simulink model "playback_data"  (R2015a)
settings: Solver=FixedStepDiscrete  SolverMode=SingleTasking  StartTime=44  StopTime=72  FixedStep=sample_time  RelTol=1e-3
undefined symbols (not defined in the file or in its folder): A_kalman_no_position, A_kalman_transverse, A_kalman_vertical, A_lpf_10hz_05d, A_lpf_accelerometer, A_lpf_fourbar_angles, A_lpf_imu, A_lpf_lateral_angle, B1_lpf_10hz_05d, B1_lpf_accelerometer, B1_lpf_fourbar_angles, B1_lpf_imu, B1_lpf_lateral_angle, B2_lpf_10hz_05d, B2_lpf_accelerometer, B2_lpf_fourbar_angles, B2_lpf_imu, B2_lpf_lateral_angle, B_dx_versus_x0, B_kalman_no_position, B_kalman_transverse, B_kalman_vertical, backwards_K_sag_of_t, backwards_P_sag_of_t, boom_mount_angle, C_kalman_no_position, C_kalman_transverse, C_kalman_vertical, com_leg_motor, com_torso, contact_threshold, control_start_time, d_ankle_to_foot, d_vertical_boom_com_offset, d_vertical_com, desired_com_forward_velocity, desired_com_lateral_velocity, desired_initial_leg_roll_left, desired_initial_leg_roll_right, desired_standing_torso_pitch, desired_standing_torso_roll, desired_standing_z, desired_torso_pitch, desired_torso_roll, Discrete, enable_bouncing, fcut_contact, fdesignblkfcn, forward_dx_of_dxstar, forward_x_of_dxstar, g, gcbh, h_boom, HIP_MTR_MAX_CONT_TORQUE, HIP_MTR_MAX_TORQUE, i_leg_motor, i_robot, i_torso, initial_dx_estimate, initial_dx_takeoff_history ... (+82)
libraries: simulink x23, ctrlSharedLib x4, dsparch4 x3, dspfdesign x1
(part 3 of 6)

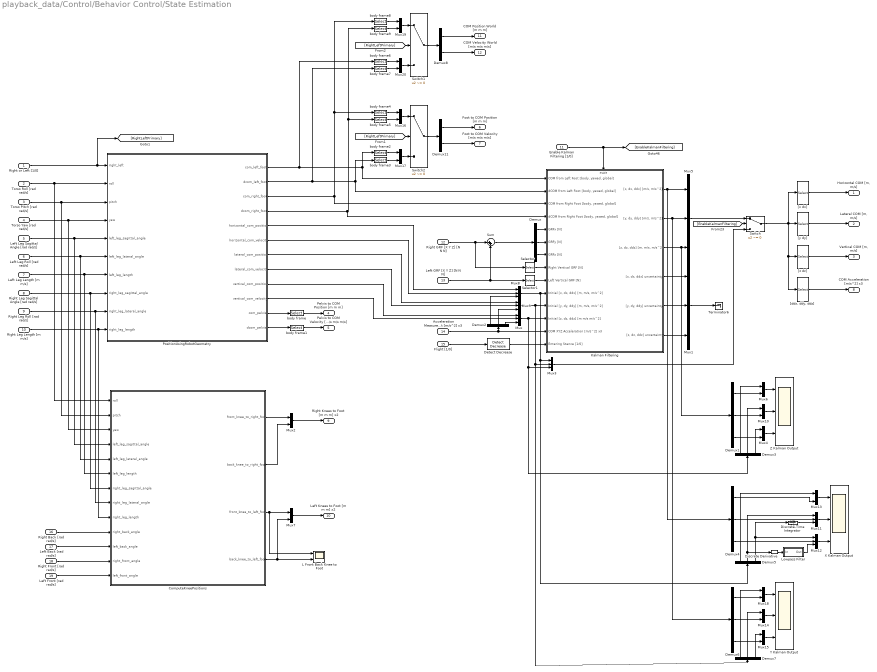
== system playback_data/Control/Behavior Control/State Estimation ==
  Right or Left [1/0] : Inport
  Torso Roll [rad rad/s] : Inport  Port=2
  Torso Pitch [rad rad/s] : Inport  Port=3
  Torso Yaw [rad rad/s] : Inport  Port=4
  Left Leg Sagittal Angle [rad rad/s] : Inport  Port=5
  Left Leg Roll [rad rad/s] : Inport  Port=6
  Left Leg Length [m m/s] : Inport  Port=7
  Right Leg Sagittal Angle [rad rad/s] : Inport  Port=8
  Right Leg Roll [rad rad/s] : Inport  Port=9
  Right Leg Length [m m/s] : Inport  Port=10
  Enable Kalman Filtering [1/0] : Inport  Port=11
  Right GRF [X Y Z] [N N N] : Inport  Port=12
  Left GRF [X Y Z] [N N N] : Inport  Port=13
  " Acceleration Measurement [m/s^2] x3" : Inport  Port=14
  Flight [1/0] : Inport  Port=15
  Right Back [rad rad/s] : Inport  Port=16
  Left Back [rad rad/s] : Inport  Port=17
  Right Front [rad rad/s] : Inport  Port=18
  Left Front [rad rad/s] : Inport  Port=19
  ComputeKneePositions : MATLAB Function  TreatAsAtomicUnit=on
  Demux{,1..7} (8 alike) : Demux  Outputs=3
  Demux11 : Demux  Outputs=2
  Demux8 : Demux  Outputs=2
  Detect Decrease : simulink/Logic and Bit Operations/Detect Decrease  vinit=0.0  InputProcessing=Inherited  OutDataTypeStr=boolean
  Discrete Derivative : simulink/Discrete/Discrete Derivative  gainval=1.0  ICPrevScaledInput=0.0  InputProcessing=Inherited  OutMin=[]  OutMax=[]  OutDataType=fixdt(1, 16)  OutScaling=2^-10  DoSatur=off
  Discrete-Time Integrator : DiscreteIntegrator  InitialConditionSetting=State (most efficient)  SampleTime=-1
  Kalman Filtering : Subsystem
  L Front Back Knee to Foot : Scope  NumInputPorts=2
      settings: YMin=-0.425~-0.5  YMax=-0.025~0.3  SaveName=ScopeData44  SampleInput=on
  Lowpass Filter : Subsystem  DialogController=fdesignblkfcn  InitFcn=fdesignblkfcn(gcbh, {'InitFcn'});  mask(Lowpass Filter){}
      mask help: Design a lowpass filter
      settings: CopyFcn=fdesignblkfcn(gcbh, {'CopyFcn'});
      mask Help: helpview(mapfilelocation('dsp'), 'dsplowpassfilter');
      mask Display: disp('Lowpass')
  Mux{,1,3,5,8..9,11..12} (8 alike) : Mux  Inputs=3
  Mux{2,4,6..7,10,13..20} (13 alike) : Mux  Inputs=2
  PositionUsingRobotGeometry : MATLAB Function  TreatAsAtomicUnit=on
  Selector : Selector  InputPortWidth=3  Indices=[3]
  Selector1 : Selector  InputPortWidth=3  Indices=[3]
  Sum : Sum  Inputs=|++
  Switch : Switch  Criteria=u2 ~= 0
  Switch1 : Switch  Criteria=u2 ~= 0
  Switch2 : Switch  Criteria=u2 ~= 0
  Terminator6 : Terminator
  X Kalman Output : Scope  NumInputPorts=3
      settings: TimeRange=3.774467455621291  YMin=-0.07~-1.4~-40  YMax=0.08~0.9~65  SaveName=ScopeData29  SampleInput=on
  Y Kalman Output : Scope  NumInputPorts=3
      settings: TimeRange=39.999  YMin=0.05~-0.7~-2  YMax=0.18~1.1~3.5  SaveName=ScopeData30  SampleInput=on
  Z Kalman Output : Scope  NumInputPorts=3
      settings: TimeRange=3.175000000000004  YMin=0~-0.04~-0.7  YMax=0.9~0.035~0.6  SaveName=ScopeData27  SampleInput=on
  "[ddx, ddy, ddz]" : Selector  InputPortWidth=9  Indices=[3 6 9]
  "[x dx]" : Selector  InputPortWidth=9  Indices=[1 2]
  "[y dy]" : Selector  InputPortWidth=9  Indices=[4 5]
  "[z dz]" : Selector  InputPortWidth=9  Indices=[7 8]
  body frame : Selector  InputPortWidth=9  Indices=[1 2 3]
  body frame1 : Selector  InputPortWidth=9  Indices=[1 2 3]
  body frame{2..5} (4 alike) : Selector  InputPortWidth=9  Indices=[4 5 6]
  body frame{6..9} (4 alike) : Selector  InputPortWidth=9  Indices=[7 8 9]
  "Horizontal COM [m, m/s]" : Outport
  "Lateral COM [m, m/s]" : Outport  Port=2
  "Vertical COM [m, m/s]" : Outport  Port=3
  Pelvis to COM Position [m m m] : Outport  Port=4
  Pelvis to COM Velocity [m/s m/s m/s] : Outport  Port=5
  Foot to COM Position [m m m] : Outport  Port=6
  Foot to COM Velocity [m/s m/s m/s] : Outport  Port=7
  COM Acceleration [m/s^2] x3 : Outport  Port=8
  Right Knees to Foot [m m m] x2 : Outport  Port=9
  Left Knees to Foot [m m m] x2 : Outport  Port=10
  COM Position World [m m m] : Outport  Port=11  PortDimensions=3
  COM Velocity World [m/s m/s m/s] : Outport  Port=12  PortDimensions=3
  wires:
  Lowpass Filter/1(Out) -> Mux12/3
  Discrete Derivative/1 -> Lowpass Filter/1(In)
  Discrete-Time Integrator/1 -> Mux11/3
  Demux5/3 -> Mux12/1, Discrete-Time Integrator/1
  Demux5/2 -> Mux11/1, Discrete Derivative/1
  Demux5/1 -> Mux13/1
  Demux4/3 -> Mux12/2
  Mux11/1 -> X Kalman Output/2
  Demux4/1 -> Mux13/2
  Demux4/2 -> Mux11/2
  Mux13/1 -> X Kalman Output/1
  Mux12/1 -> X Kalman Output/3
  Mux9/1 -> Mux3/2, Demux7/1, Kalman Filtering/11("Initial [y, dy, ddy] [m, m/s, m/s^2]")
  Mux8/1 -> Mux3/1, Demux5/1, Kalman Filtering/10("Initial [x, dx, ddx] [m, m/s, m/s^2]")
  "[ddx, ddy, ddz]"/1 -> COM Acceleration [m/s^2] x3/1
  Mux3/1 -> Switch/3
  Demux2/2 -> Mux9/3
  Demux2/1 -> Mux8/3
  Demux2/3 -> Mux/3
  " Acceleration Measurement [m/s^2] x3"/1 -> Demux2/1, Kalman Filtering/13(COM XYZ Acceleration [m/s^2] x3)
  PositionUsingRobotGeometry/5(horizontal_com_position) -> Mux8/1
  Left Leg Sagittal Angle [rad rad/s]/1 -> PositionUsingRobotGeometry/5(left_leg_sagittal_angle), ComputeKneePositions/4(left_leg_sagittal_angle)
  Left Leg Roll [rad rad/s]/1 -> PositionUsingRobotGeometry/6(left_leg_lateral_angle), ComputeKneePositions/5(left_leg_lateral_angle)
  Left Leg Length [m m/s]/1 -> PositionUsingRobotGeometry/7(left_leg_length), ComputeKneePositions/6(left_leg_length)
  Right Leg Sagittal Angle [rad rad/s]/1 -> PositionUsingRobotGeometry/8(right_leg_sagittal_angle), ComputeKneePositions/7(right_leg_sagittal_angle)
  Right Leg Roll [rad rad/s]/1 -> ComputeKneePositions/8(right_leg_lateral_angle), PositionUsingRobotGeometry/9(right_leg_lateral_angle)
  Right Leg Length [m m/s]/1 -> ComputeKneePositions/9(right_leg_length), PositionUsingRobotGeometry/10(right_leg_length)
  Right or Left [1/0]/1 -> [RightLeftPrimary], PositionUsingRobotGeometry/1(right_left)
  Torso Roll [rad rad/s]/1 -> PositionUsingRobotGeometry/2(roll), ComputeKneePositions/1(roll)
  Torso Yaw [rad rad/s]/1 -> PositionUsingRobotGeometry/4(yaw), ComputeKneePositions/3(yaw)
  Torso Pitch [rad rad/s]/1 -> PositionUsingRobotGeometry/3(pitch), ComputeKneePositions/2(pitch)
  Mux5/1 -> Switch/1
  Selector/1 -> Kalman Filtering/8(Right Vertical GRF [N])
  Selector1/1 -> Kalman Filtering/9(Left Vertical GRF [N])
  Left GRF [X Y Z] [N N N]/1 -> Sum/2, Selector1/1
  Right GRF [X Y Z] [N N N]/1 -> Selector/1, Sum/1
  Sum/1 -> Demux/1
  Enable Kalman Filtering [1/0]/1 -> Kalman Filtering/Enable, [EnableKalmanFiltering]
  Demux/1 -> Kalman Filtering/5(GRFx [N])
  Mux1/1 -> Terminator6/1
  PositionUsingRobotGeometry/12(dcom_pelvis) -> body frame1/1
  PositionUsingRobotGeometry/11(com_pelvis) -> body frame/1
  "[x dx]"/1 -> "Horizontal COM [m, m/s]"/1
  body frame/1 -> Pelvis to COM Position [m m m]/1
  body frame1/1 -> Pelvis to COM Velocity [m/s m/s m/s]/1
  PositionUsingRobotGeometry/7(lateral_com_position) -> Mux9/1
  "[z dz]"/1 -> "Vertical COM [m, m/s]"/1
  Switch/1 -> "[x dx]"/1, "[y dy]"/1, "[z dz]"/1, "[ddx, ddy, ddz]"/1
  "[y dy]"/1 -> "Lateral COM [m, m/s]"/1
  Demux/3 -> Kalman Filtering/7(GRFz [N])
  Demux/2 -> Kalman Filtering/6(GRFy [N])
  Kalman Filtering/1("[x, dx, ddx] [m/s, m/s^2]") -> Mux5/1, Demux4/1
  Kalman Filtering/3("[z, dz, ddz] [m, m/s, m/s^2]") -> Demux1/1, Mux5/3
  Kalman Filtering/2("[y, dy, ddy] [m/s, m/s^2]") -> Demux6/1, Mux5/2
  Kalman Filtering/5("[y, dy, ddy] uncertainty") -> Mux1/2
  Kalman Filtering/4("[x, dx, ddx] uncertainty") -> Mux1/1
  Kalman Filtering/6("[z, dz, ddz] uncertainty") -> Mux1/3
  PositionUsingRobotGeometry/9(vertical_com_position) -> Mux/1
  PositionUsingRobotGeometry/10(vertical_com_velocity) -> Mux/2
  Mux/1 -> Mux3/3, Demux3/1, Kalman Filtering/12("Initial [z, dz, ddz] [m m/s m/s^2]")
  PositionUsingRobotGeometry/8(lateral_com_velocity) -> Mux9/2
  PositionUsingRobotGeometry/6(horizontal_com_velocity) -> Mux8/2
  [RightLeftPrimary] -> Switch2/2
  Mux17/1 -> Switch2/3
  Mux16/1 -> Switch2/1
  Switch2/1 -> Demux11/1
  Demux11/2 -> Foot to COM Velocity [m/s m/s m/s]/1
  Demux11/1 -> Foot to COM Position [m m m]/1
  body frame2/1 -> Mux17/1
  body frame3/1 -> Mux17/2
  body frame5/1 -> Mux16/2
  body frame4/1 -> Mux16/1
  Flight [1/0]/1 -> Detect Decrease/1
  Detect Decrease/1 -> Kalman Filtering/14(Entering Stance [1/0])
  Mux4/1 -> Z Kalman Output/3
  Mux6/1 -> Z Kalman Output/1
  Demux1/2 -> Mux10/2
  Demux1/1 -> Mux6/2
  Mux10/1 -> Z Kalman Output/2
  Demux1/3 -> Mux4/2
  Demux3/1 -> Mux6/1
  Demux3/2 -> Mux10/1
  Demux3/3 -> Mux4/1
  Mux15/1 -> Y Kalman Output/3
  Mux18/1 -> Y Kalman Output/1
  Demux6/2 -> Mux14/2
  Demux6/1 -> Mux18/2
  Mux14/1 -> Y Kalman Output/2
  Demux6/3 -> Mux15/2
  Demux7/1 -> Mux18/1
  Demux7/2 -> Mux14/1
  Demux7/3 -> Mux15/1
  ComputeKneePositions/1(front_knee_to_right_foot) -> Mux2/1
  ComputeKneePositions/2(back_knee_to_right_foot) -> Mux2/2
  ComputeKneePositions/3(front_knee_to_left_foot) -> L Front Back Knee to Foot/1, Mux7/1
  ComputeKneePositions/4(back_knee_to_left_foot) -> L Front Back Knee to Foot/2, Mux7/2
  Mux2/1 -> Right Knees to Foot [m m m] x2/1
  Mux7/1 -> Left Knees to Foot [m m m] x2/1
  Left Front [rad rad/s]/1 -> ComputeKneePositions/13(left_front_angle)
  Right Front [rad rad/s]/1 -> ComputeKneePositions/12(right_front_angle)
  Left Back [rad rad/s]/1 -> ComputeKneePositions/11(left_back_angle)
  Right Back [rad rad/s]/1 -> ComputeKneePositions/10(right_back_angle)
  [EnableKalmanFiltering] -> Switch/2
  PositionUsingRobotGeometry/1(com_left_foot) -> body frame6/1, body frame2/1, Kalman Filtering/1("COM from Left Foot [body, yawed, global]")
  PositionUsingRobotGeometry/2(dcom_left_foot) -> body frame7/1, body frame3/1, Kalman Filtering/2("dCOM from Left Foot [body, yawed, global]")
  PositionUsingRobotGeometry/3(com_right_foot) -> body frame8/1, body frame4/1, Kalman Filtering/3("COM from Right Foot [body, yawed, global]")
  PositionUsingRobotGeometry/4(dcom_right_foot) -> Kalman Filtering/4("dCOM from Right Foot [body, yawed, global]"), body frame9/1, body frame5/1
  [RightLeftPrimary] -> Switch1/2
  Mux20/1 -> Switch1/3
  Mux19/1 -> Switch1/1
  Switch1/1 -> Demux8/1
  Demux8/2 -> COM Velocity World [m/s m/s m/s]/1
  Demux8/1 -> COM Position World [m m m]/1
  body frame6/1 -> Mux20/1
  body frame7/1 -> Mux20/2
  body frame9/1 -> Mux19/2
  body frame8/1 -> Mux19/1

== system playback_data/Control/Behavior Control/Atrias Swing control/Back//Front PD ==
  Desired Position [rad] [back front] : Inport
  Desired Velocity [rad/s] [back front] : Inport  Port=2
  Measured Position [rad] [back front] : Inport  Port=3
  Back / Front PositionTracking : Scope  NumInputPorts=2
      settings: YMin=3.725~-1  YMax=4.05~0.9  SaveName=ScopeData6  SampleInput=on
  Feedback / Feedforward : Scope  NumInputPorts=2
      settings: YMin=-2~-3  YMax=4.5~3  SaveName=ScopeData45  SampleInput=on
  Feedforward Gain : Gain
  Kp_SEA_Trajectory : Constant  Value=kp_velocity_swing_trajectory
  Mux13 : Mux  Inputs=2
  Mux2 : Mux  Inputs=2
  Product1 : Product
  Selector : Selector  InputPortWidth=2  Indices=[1]
  Selector1 : Selector  InputPortWidth=2  Indices=[1]
  Selector4 : Selector  InputPortWidth=2  Indices=[2]
  Selector5 : Selector  InputPortWidth=2  Indices=[2]
  Sum7 : Sum  Inputs=|+-
  Sum9 : Sum
  Commanded Velocity [rad/s] [back front] : Outport
  wires:
  Feedforward Gain/1 -> Sum9/2, Feedback / Feedforward/2
  Desired Velocity [rad/s] [back front]/1 -> Feedforward Gain/1
  Selector4/1 -> Mux2/1
  Selector5/1 -> Mux2/2
  Selector1/1 -> Mux13/2
  Selector/1 -> Mux13/1
  Mux2/1 -> Back / Front PositionTracking/2
  Desired Position [rad] [back front]/1 -> Sum7/1, Selector1/1, Selector5/1
  Mux13/1 -> Back / Front PositionTracking/1
  Product1/1 -> Sum9/1, Feedback / Feedforward/1
  Sum7/1 -> Product1/1
  Measured Position [rad] [back front]/1 -> Sum7/2, Selector/1, Selector4/1
  Sum9/1 -> Commanded Velocity [rad/s] [back front]/1
  Kp_SEA_Trajectory/1 -> Product1/2

== system playback_data/Control/Behavior Control/Force Estimation/Leg Force Measurements ==
  q : Inport
  Leg Width Right/Left [m m] : Inport  Port=2
  Leg Length Right/Left [m m] : Inport  Port=3
  Demux : Demux  Outputs=2
  Demux1 : Demux  Outputs=2
  Demux2 : Demux
  Divide{1..4} (4 alike) : Product  Inputs=*/
  Gain : Gain  Commented=on  Gain=k_sea_low
  Mux : Mux
  Nonlinear Spring Force : MATLAB Function  TreatAsAtomicUnit=on
  Sum{1..3,6} (4 alike) : Sum  Inputs=-+|
  Sum4 : Sum  Inputs=-|+
  Sum5 : Sum  Inputs=-|+
  Sum7 : Sum  Inputs=+|+
  Sum8 : Sum  Inputs=+|+
  backGearL : Selector  InputPortWidth=13  Indices=[6]
  backGearR : Selector  InputPortWidth=13  Indices=[2]
  backJointL : Selector  InputPortWidth=13  Indices=[5]
  backJointR : Selector  InputPortWidth=13  Indices=[1]
  frontGearL : Selector  InputPortWidth=13  Indices=[8]
  frontGearR : Selector  InputPortWidth=13  Indices=[4]
  frontJointL : Selector  InputPortWidth=13  Indices=[7]
  frontJointR : Selector  InputPortWidth=13  Indices=[3]
  Right Leg Torque [Nm] : Outport
  Left Leg Torque [Nm] : Outport  Port=2
  Right Leg Axial Force [N] : Outport  Port=3
  Left Leg Axial Force [N] : Outport  Port=4
  Right Leg Orthogonal Force [N] : Outport  Port=5
  Left Leg Orthogonal Force [N] : Outport  Port=6
  wires:
  Sum3/1 -> Mux/4
  Sum2/1 -> Mux/3
  backJointL/1 -> Sum2/1
  frontGearL/1 -> Sum3/2
  frontJointL/1 -> Sum3/1
  backGearL/1 -> Sum2/2
  Sum6/1 -> Mux/1
  Sum1/1 -> Mux/2
  backJointR/1 -> Sum6/1
  frontGearR/1 -> Sum1/2
  frontJointR/1 -> Sum1/1
  backGearR/1 -> Sum6/2
  q/1 -> backGearR/1, backJointL/1, frontJointL/1, frontGearL/1, backGearL/1, frontGearR/1, frontJointR/1, backJointR/1
  Demux2/1 -> Sum4/1, Sum7/1
  Demux2/2 -> Sum7/2, Sum4/2
  Demux2/4 -> Sum5/2, Sum8/2
  Sum4/1 -> Divide1/1
  Sum5/1 -> Divide2/1
  Leg Width Right/Left [m m]/1 -> Demux/1
  Demux/1 -> Divide1/2
  Demux/2 -> Divide2/2
  Divide1/1 -> Right Leg Axial Force [N]/1
  Divide2/1 -> Left Leg Axial Force [N]/1
  Demux2/3 -> Sum8/1, Sum5/1
  Sum7/1 -> Divide3/1, Right Leg Torque [Nm]/1
  Sum8/1 -> Divide4/1, Left Leg Torque [Nm]/1
  Demux1/1 -> Divide3/2
  Demux1/2 -> Divide4/2
  Leg Length Right/Left [m m]/1 -> Demux1/1
  Divide3/1 -> Right Leg Orthogonal Force [N]/1
  Divide4/1 -> Left Leg Orthogonal Force [N]/1
  Mux/1 -> Nonlinear Spring Force/1(deflections)
  Nonlinear Spring Force/1(tau_sea) -> Demux2/1

== system playback_data/Control/Behavior Control/Force Estimation/Leg Plane GRF ==
  Axial Force [N] : Inport
  Orthogonal Force [N] : Inport  Port=2
  Torso Pitch [rad] : Inport  Port=3
  Leg Angle [rad] : Inport  Port=4
  Gain : Gain  Gain=-1
  Product : Product
  Product1 : Product
  Sum : Sum  Inputs=++|
  Sum1 : Sum  Inputs=+|+
  Trigonometric Function : Trigonometry  Operator=cos
  Trigonometric Function1 : Trigonometry
  Vertical Force [N] : Outport
  wires:
  Product1/1 -> Sum1/2
  Sum1/1 -> Vertical Force [N]/1
  Trigonometric Function1/1 -> Product1/2
  Orthogonal Force [N]/1 -> Product1/1
  Axial Force [N]/1 -> Product/1
  Leg Angle [rad]/1 -> Sum/2
  Torso Pitch [rad]/1 -> Sum/1
  Trigonometric Function/1 -> Product/2
  Product/1 -> Gain/1
  Sum/1 -> Trigonometric Function/1, Trigonometric Function1/1
  Gain/1 -> Sum1/1

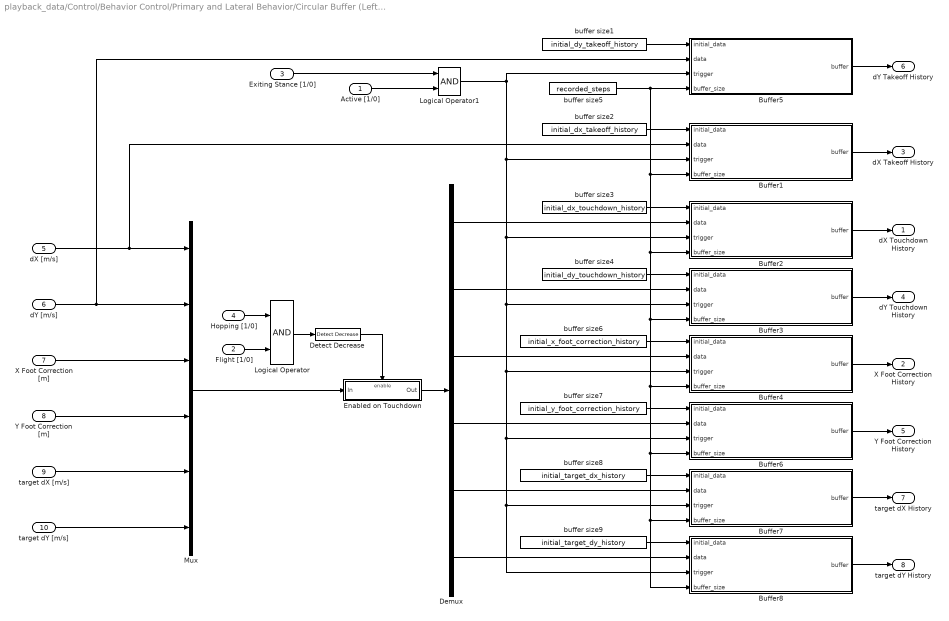
== system playback_data/Control/Behavior Control/Primary and Lateral Behavior/Circular Buffer (Left Foot) ==
  Active [1/0] : Inport
  Flight [1/0] : Inport  Port=2
  Exiting Stance [1/0] : Inport  Port=3
  Hopping [1/0] : Inport  Port=4
  dX [m/s] : Inport  Port=5
  dY [m/s] : Inport  Port=6
  X Foot Correction [m] : Inport  Port=7
  Y Foot Correction [m] : Inport  Port=8
  target dX [m/s] : Inport  Port=9
  target dY [m/s] : Inport  Port=10
  Buffer1 : MATLAB Function  TreatAsAtomicUnit=on  SystemSampleTime=sample_time
  Buffer2 : MATLAB Function  TreatAsAtomicUnit=on  SystemSampleTime=sample_time
  Buffer3 : MATLAB Function  TreatAsAtomicUnit=on  SystemSampleTime=sample_time
  Buffer4 : MATLAB Function  TreatAsAtomicUnit=on  SystemSampleTime=sample_time
  Buffer5 : MATLAB Function  TreatAsAtomicUnit=on  SystemSampleTime=sample_time
  Buffer6 : MATLAB Function  TreatAsAtomicUnit=on  SystemSampleTime=sample_time
  Buffer7 : MATLAB Function  TreatAsAtomicUnit=on  SystemSampleTime=sample_time
  Buffer8 : MATLAB Function  TreatAsAtomicUnit=on  SystemSampleTime=sample_time
  Demux : Demux  Outputs=6
  Detect Decrease : simulink/Logic and Bit Operations/Detect Decrease  vinit=0.0  InputProcessing=Inherited  OutDataTypeStr=boolean
  Enabled on Touchdown : Subsystem  TreatAsAtomicUnit=on
  Logical Operator : Logic  AllPortsSameDT=off  OutDataTypeStr=boolean
  Logical Operator1 : Logic  AllPortsSameDT=off  OutDataTypeStr=boolean
  Mux : Mux  Inputs=6
  buffer size1 : Constant  Value=initial_dy_takeoff_history
  buffer size2 : Constant  Value=initial_dx_takeoff_history
  buffer size3 : Constant  Value=initial_dx_touchdown_history
  buffer size4 : Constant  Value=initial_dy_touchdown_history
  buffer size5 : Constant  Value=recorded_steps
  buffer size6 : Constant  Value=initial_x_foot_correction_history
  buffer size7 : Constant  Value=initial_y_foot_correction_history
  buffer size8 : Constant  Value=initial_target_dx_history
  buffer size9 : Constant  Value=initial_target_dy_history
  "dX Touchdown History " : Outport
  X Foot Correction History : Outport  Port=2
  dX Takeoff History : Outport  Port=3
  "dY Touchdown History " : Outport  Port=4
  Y Foot Correction History : Outport  Port=5
  dY Takeoff History : Outport  Port=6
  target dX History : Outport  Port=7
  target dY History : Outport  Port=8
  wires:
  Exiting Stance [1/0]/1 -> Logical Operator1/1
  Active [1/0]/1 -> Logical Operator1/2
  buffer size9/1 -> Buffer8/1(initial_data)
  buffer size8/1 -> Buffer7/1(initial_data)
  buffer size7/1 -> Buffer6/1(initial_data)
  buffer size6/1 -> Buffer4/1(initial_data)
  buffer size4/1 -> Buffer3/1(initial_data)
  buffer size3/1 -> Buffer2/1(initial_data)
  buffer size2/1 -> Buffer1/1(initial_data)
  buffer size1/1 -> Buffer5/1(initial_data)
  Buffer2/1(buffer) -> "dX Touchdown History "/1
  Detect Decrease/1 -> Enabled on Touchdown/Enable
  Buffer4/1(buffer) -> X Foot Correction History/1
  Buffer1/1(buffer) -> dX Takeoff History/1
  Demux/1 -> Buffer2/2(data)
  Demux/3 -> Buffer4/2(data)
  X Foot Correction [m]/1 -> Mux/3
  Buffer3/1(buffer) -> "dY Touchdown History "/1
  Buffer6/1(buffer) -> Y Foot Correction History/1
  Demux/2 -> Buffer3/2(data)
  Buffer5/1(buffer) -> dY Takeoff History/1
  Y Foot Correction [m]/1 -> Mux/4
  Demux/4 -> Buffer6/2(data)
  target dX [m/s]/1 -> Mux/5
  Buffer7/1(buffer) -> target dX History/1
  Buffer8/1(buffer) -> target dY History/1
  buffer size5/1 -> Buffer1/4(buffer_size), Buffer2/4(buffer_size), Buffer3/4(buffer_size), Buffer4/4(buffer_size), Buffer6/4(buffer_size), Buffer8/4(buffer_size), Buffer7/4(buffer_size), Buffer5/4(buffer_size)
  Demux/6 -> Buffer8/2(data)
  Demux/5 -> Buffer7/2(data)
  target dY [m/s]/1 -> Mux/6
  Logical Operator1/1 -> Buffer5/3(trigger), Buffer1/3(trigger), Buffer2/3(trigger), Buffer3/3(trigger), Buffer4/3(trigger), Buffer6/3(trigger), Buffer8/3(trigger), Buffer7/3(trigger)
  Hopping [1/0]/1 -> Logical Operator/1
  dY [m/s]/1 -> Buffer5/2(data), Mux/2
  dX [m/s]/1 -> Buffer1/2(data), Mux/1
  Flight [1/0]/1 -> Logical Operator/2
  Logical Operator/1 -> Detect Decrease/1
  Mux/1 -> Enabled on Touchdown/1(In)
  Enabled on Touchdown/1(Out) -> Demux/1

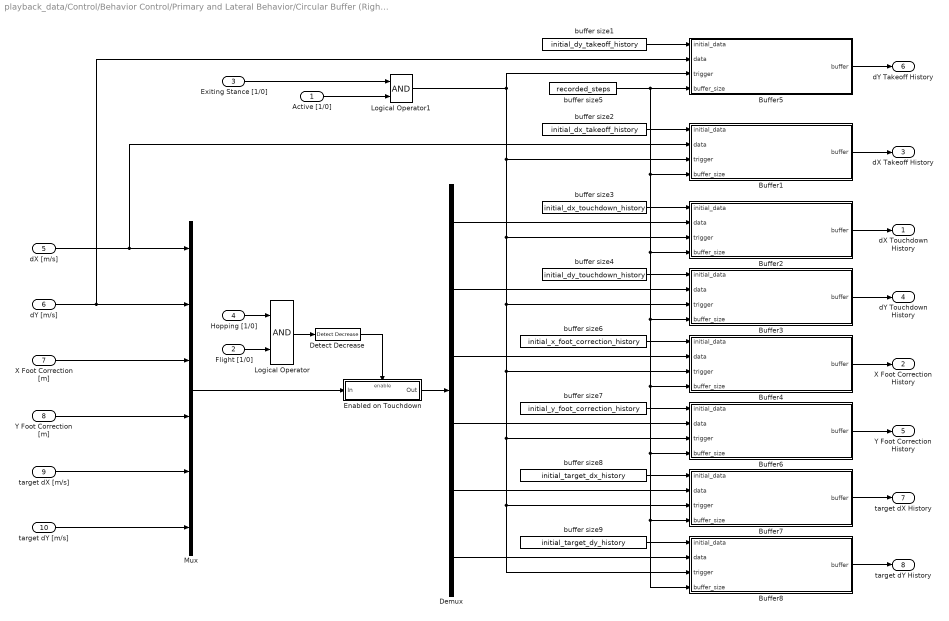
== system playback_data/Control/Behavior Control/Primary and Lateral Behavior/Circular Buffer (Right Foot) ==
  Active [1/0] : Inport
  Flight [1/0] : Inport  Port=2
  Exiting Stance [1/0] : Inport  Port=3
  Hopping [1/0] : Inport  Port=4
  dX [m/s] : Inport  Port=5
  dY [m/s] : Inport  Port=6
  X Foot Correction [m] : Inport  Port=7
  Y Foot Correction [m] : Inport  Port=8
  target dX [m/s] : Inport  Port=9
  target dY [m/s] : Inport  Port=10
  Buffer1 : MATLAB Function  TreatAsAtomicUnit=on  SystemSampleTime=sample_time
  Buffer2 : MATLAB Function  TreatAsAtomicUnit=on  SystemSampleTime=sample_time
  Buffer3 : MATLAB Function  TreatAsAtomicUnit=on  SystemSampleTime=sample_time
  Buffer4 : MATLAB Function  TreatAsAtomicUnit=on  SystemSampleTime=sample_time
  Buffer5 : MATLAB Function  TreatAsAtomicUnit=on  SystemSampleTime=sample_time
  Buffer6 : MATLAB Function  TreatAsAtomicUnit=on  SystemSampleTime=sample_time
  Buffer7 : MATLAB Function  TreatAsAtomicUnit=on  SystemSampleTime=sample_time
  Buffer8 : MATLAB Function  TreatAsAtomicUnit=on  SystemSampleTime=sample_time
  Demux : Demux  Outputs=6
  Detect Decrease : simulink/Logic and Bit Operations/Detect Decrease  vinit=0.0  InputProcessing=Inherited  OutDataTypeStr=boolean
  Enabled on Touchdown : Subsystem  TreatAsAtomicUnit=on
  Logical Operator : Logic  AllPortsSameDT=off  OutDataTypeStr=boolean
  Logical Operator1 : Logic  AllPortsSameDT=off  OutDataTypeStr=boolean
  Mux : Mux  Inputs=6
  buffer size1 : Constant  Value=initial_dy_takeoff_history
  buffer size2 : Constant  Value=initial_dx_takeoff_history
  buffer size3 : Constant  Value=initial_dx_touchdown_history
  buffer size4 : Constant  Value=initial_dy_touchdown_history
  buffer size5 : Constant  Value=recorded_steps
  buffer size6 : Constant  Value=initial_x_foot_correction_history
  buffer size7 : Constant  Value=initial_y_foot_correction_history
  buffer size8 : Constant  Value=initial_target_dx_history
  buffer size9 : Constant  Value=initial_target_dy_history
  "dX Touchdown History " : Outport
  X Foot Correction History : Outport  Port=2
  dX Takeoff History : Outport  Port=3
  "dY Touchdown History " : Outport  Port=4
  Y Foot Correction History : Outport  Port=5
  dY Takeoff History : Outport  Port=6
  target dX History : Outport  Port=7
  target dY History : Outport  Port=8
  wires:
  Active [1/0]/1 -> Logical Operator1/2
  Exiting Stance [1/0]/1 -> Logical Operator1/1
  Enabled on Touchdown/1(Out) -> Demux/1
  Mux/1 -> Enabled on Touchdown/1(In)
  Logical Operator/1 -> Detect Decrease/1
  Flight [1/0]/1 -> Logical Operator/2
  dX [m/s]/1 -> Mux/1, Buffer1/2(data)
  dY [m/s]/1 -> Mux/2, Buffer5/2(data)
  Hopping [1/0]/1 -> Logical Operator/1
  Logical Operator1/1 -> Buffer7/3(trigger), Buffer8/3(trigger), Buffer6/3(trigger), Buffer4/3(trigger), Buffer3/3(trigger), Buffer2/3(trigger), Buffer1/3(trigger), Buffer5/3(trigger)
  target dY [m/s]/1 -> Mux/6
  Demux/5 -> Buffer7/2(data)
  Demux/6 -> Buffer8/2(data)
  buffer size5/1 -> Buffer5/4(buffer_size), Buffer7/4(buffer_size), Buffer8/4(buffer_size), Buffer6/4(buffer_size), Buffer4/4(buffer_size), Buffer3/4(buffer_size), Buffer2/4(buffer_size), Buffer1/4(buffer_size)
  Buffer8/1(buffer) -> target dY History/1
  Buffer7/1(buffer) -> target dX History/1
  target dX [m/s]/1 -> Mux/5
  Demux/4 -> Buffer6/2(data)
  Y Foot Correction [m]/1 -> Mux/4
  Buffer5/1(buffer) -> dY Takeoff History/1
  Demux/2 -> Buffer3/2(data)
  Buffer6/1(buffer) -> Y Foot Correction History/1
  Buffer3/1(buffer) -> "dY Touchdown History "/1
  X Foot Correction [m]/1 -> Mux/3
  Demux/3 -> Buffer4/2(data)
  Demux/1 -> Buffer2/2(data)
  Buffer1/1(buffer) -> dX Takeoff History/1
  Buffer4/1(buffer) -> X Foot Correction History/1
  Detect Decrease/1 -> Enabled on Touchdown/Enable
  Buffer2/1(buffer) -> "dX Touchdown History "/1
  buffer size1/1 -> Buffer5/1(initial_data)
  buffer size2/1 -> Buffer1/1(initial_data)
  buffer size3/1 -> Buffer2/1(initial_data)
  buffer size4/1 -> Buffer3/1(initial_data)
  buffer size6/1 -> Buffer4/1(initial_data)
  buffer size7/1 -> Buffer6/1(initial_data)
  buffer size8/1 -> Buffer7/1(initial_data)
  buffer size9/1 -> Buffer8/1(initial_data)

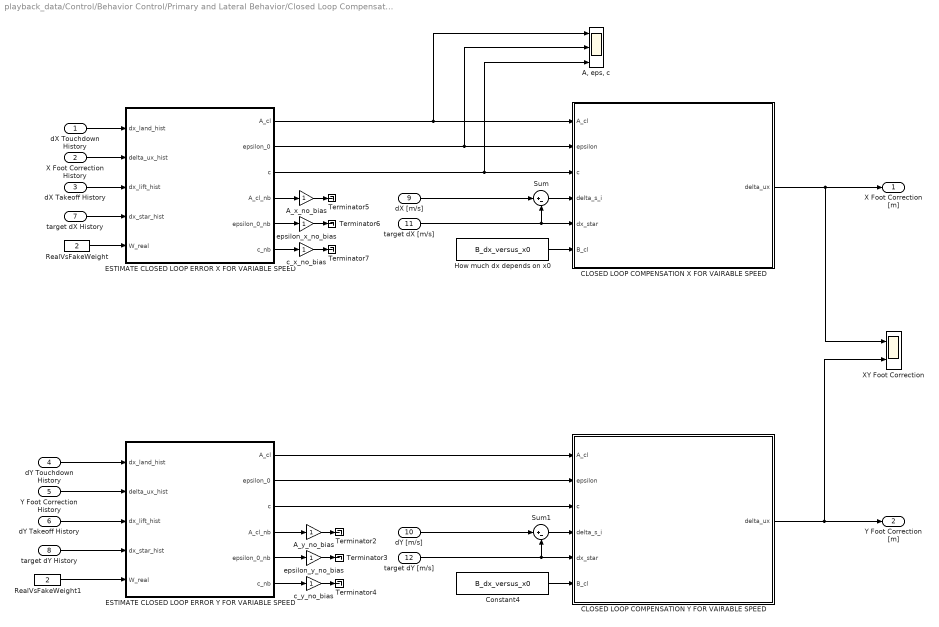
== system playback_data/Control/Behavior Control/Primary and Lateral Behavior/Closed Loop Compensation (Left Foot) ==
  dX Touchdown History : Inport
  X Foot Correction History : Inport  Port=2
  dX Takeoff History : Inport  Port=3
  dY Touchdown History : Inport  Port=4
  Y Foot Correction History : Inport  Port=5
  dY Takeoff History : Inport  Port=6
  target dX History : Inport  Port=7
  target dY History : Inport  Port=8
  dX [m/s] : Inport  Port=9
  dY [m/s] : Inport  Port=10
  target dX [m/s] : Inport  Port=11
  "target dY [m/s] " : Inport  Port=12
  "A, eps, c" : Scope  NumInputPorts=3
      settings: YMin=-1~-0.8~-5  YMax=1~1.4~5  SaveName=ScopeData56  SampleInput=on
  A_x_no_bias : Gain
  A_y_no_bias : Gain
  CLOSED LOOP COMPENSATION X FOR VAIRABLE SPEED : MATLAB Function  TreatAsAtomicUnit=on
  CLOSED LOOP COMPENSATION Y FOR VAIRABLE SPEED : MATLAB Function  TreatAsAtomicUnit=on
  Constant4 : Constant  Value=B_dx_versus_x0
  ESTIMATE CLOSED LOOP ERROR X FOR VARIABLE SPEED : MATLAB Function  TreatAsAtomicUnit=on
  ESTIMATE CLOSED LOOP ERROR Y FOR VARIABLE SPEED : MATLAB Function  TreatAsAtomicUnit=on
  How much dx depends on x0 : Constant  Value=B_dx_versus_x0
  RealVsFakeWeight : Constant  Value=2
  RealVsFakeWeight1 : Constant  Value=2
  Sum : Sum  Inputs=|+-
  Sum1 : Sum  Inputs=|+-
  Terminator{2..7} (6 alike) : Terminator
  XY Foot Correction : Scope  NumInputPorts=2
      settings: YMin=-1.75~-0.25  YMax=0.25~0.25  SaveName=ScopeData39  SampleInput=on
  c_x_no_bias : Gain
  c_y_no_bias : Gain
  epsilon_x_no_bias : Gain
  epsilon_y_no_bias : Gain
  X Foot Correction [m] : Outport
  Y Foot Correction [m] : Outport  Port=2
  wires:
  ESTIMATE CLOSED LOOP ERROR Y FOR VARIABLE SPEED/1(A_cl) -> CLOSED LOOP COMPENSATION Y FOR VAIRABLE SPEED/1(A_cl)
  ESTIMATE CLOSED LOOP ERROR Y FOR VARIABLE SPEED/2(epsilon_0) -> CLOSED LOOP COMPENSATION Y FOR VAIRABLE SPEED/2(epsilon)
  ESTIMATE CLOSED LOOP ERROR Y FOR VARIABLE SPEED/3(c) -> CLOSED LOOP COMPENSATION Y FOR VAIRABLE SPEED/3(c)
  ESTIMATE CLOSED LOOP ERROR X FOR VARIABLE SPEED/1(A_cl) -> "A, eps, c"/1, CLOSED LOOP COMPENSATION X FOR VAIRABLE SPEED/1(A_cl)
  ESTIMATE CLOSED LOOP ERROR X FOR VARIABLE SPEED/2(epsilon_0) -> CLOSED LOOP COMPENSATION X FOR VAIRABLE SPEED/2(epsilon), "A, eps, c"/2
  ESTIMATE CLOSED LOOP ERROR X FOR VARIABLE SPEED/3(c) -> CLOSED LOOP COMPENSATION X FOR VAIRABLE SPEED/3(c), "A, eps, c"/3
  ESTIMATE CLOSED LOOP ERROR Y FOR VARIABLE SPEED/6(c_nb) -> c_y_no_bias/1
  ESTIMATE CLOSED LOOP ERROR Y FOR VARIABLE SPEED/5(epsilon_0_nb) -> epsilon_y_no_bias/1
  ESTIMATE CLOSED LOOP ERROR Y FOR VARIABLE SPEED/4(A_cl_nb) -> A_y_no_bias/1
  c_y_no_bias/1 -> Terminator4/1
  epsilon_y_no_bias/1 -> Terminator3/1
  A_y_no_bias/1 -> Terminator2/1
  c_x_no_bias/1 -> Terminator7/1
  epsilon_x_no_bias/1 -> Terminator6/1
  A_x_no_bias/1 -> Terminator5/1
  ESTIMATE CLOSED LOOP ERROR X FOR VARIABLE SPEED/4(A_cl_nb) -> A_x_no_bias/1
  ESTIMATE CLOSED LOOP ERROR X FOR VARIABLE SPEED/5(epsilon_0_nb) -> epsilon_x_no_bias/1
  ESTIMATE CLOSED LOOP ERROR X FOR VARIABLE SPEED/6(c_nb) -> c_x_no_bias/1
  CLOSED LOOP COMPENSATION Y FOR VAIRABLE SPEED/1(delta_ux) -> Y Foot Correction [m]/1, XY Foot Correction/2
  CLOSED LOOP COMPENSATION X FOR VAIRABLE SPEED/1(delta_ux) -> X Foot Correction [m]/1, XY Foot Correction/1
  Sum1/1 -> CLOSED LOOP COMPENSATION Y FOR VAIRABLE SPEED/4(delta_s_i)
  dY Touchdown History/1 -> ESTIMATE CLOSED LOOP ERROR Y FOR VARIABLE SPEED/1(dx_land_hist)
  dX [m/s]/1 -> Sum/1
  dX Touchdown History/1 -> ESTIMATE CLOSED LOOP ERROR X FOR VARIABLE SPEED/1(dx_land_hist)
  dX Takeoff History/1 -> ESTIMATE CLOSED LOOP ERROR X FOR VARIABLE SPEED/3(dx_lift_hist)
  X Foot Correction History/1 -> ESTIMATE CLOSED LOOP ERROR X FOR VARIABLE SPEED/2(delta_ux_hist)
  target dX History/1 -> ESTIMATE CLOSED LOOP ERROR X FOR VARIABLE SPEED/4(dx_star_hist)
  target dX [m/s]/1 -> CLOSED LOOP COMPENSATION X FOR VAIRABLE SPEED/5(dx_star), Sum/2
  Sum/1 -> CLOSED LOOP COMPENSATION X FOR VAIRABLE SPEED/4(delta_s_i)
  How much dx depends on x0/1 -> CLOSED LOOP COMPENSATION X FOR VAIRABLE SPEED/6(B_cl)
  RealVsFakeWeight/1 -> ESTIMATE CLOSED LOOP ERROR X FOR VARIABLE SPEED/5(W_real)
  dY [m/s]/1 -> Sum1/1
  dY Takeoff History/1 -> ESTIMATE CLOSED LOOP ERROR Y FOR VARIABLE SPEED/3(dx_lift_hist)
  Y Foot Correction History/1 -> ESTIMATE CLOSED LOOP ERROR Y FOR VARIABLE SPEED/2(delta_ux_hist)
  target dY History/1 -> ESTIMATE CLOSED LOOP ERROR Y FOR VARIABLE SPEED/4(dx_star_hist)
  "target dY [m/s] "/1 -> CLOSED LOOP COMPENSATION Y FOR VAIRABLE SPEED/5(dx_star), Sum1/2
  Constant4/1 -> CLOSED LOOP COMPENSATION Y FOR VAIRABLE SPEED/6(B_cl)
  RealVsFakeWeight1/1 -> ESTIMATE CLOSED LOOP ERROR Y FOR VARIABLE SPEED/5(W_real)

== system playback_data/Control/Behavior Control/Primary and Lateral Behavior/Closed Loop Compensation (Right Foot) ==
  dX Touchdown History : Inport
  X Foot Correction History : Inport  Port=2
  dX Takeoff History : Inport  Port=3
  dY Touchdown History : Inport  Port=4
  Y Foot Correction History : Inport  Port=5
  dY Takeoff History : Inport  Port=6
  target dX History : Inport  Port=7
  target dY History : Inport  Port=8
  dX [m/s] : Inport  Port=9
  dY [m/s] : Inport  Port=10
  target dX [m/s] : Inport  Port=11
  "target dY [m/s] " : Inport  Port=12
  "A, eps, c" : Scope  NumInputPorts=3
      settings: YMin=-1~-0.8~-5  YMax=1~1.4~5  SaveName=ScopeData56  SampleInput=on
  A_x_no_bias : Gain
  A_y_no_bias : Gain
  CLOSED LOOP COMPENSATION X FOR VAIRABLE SPEED : MATLAB Function  TreatAsAtomicUnit=on
  CLOSED LOOP COMPENSATION Y FOR VAIRABLE SPEED : MATLAB Function  TreatAsAtomicUnit=on
  Constant4 : Constant  Value=B_dx_versus_x0
  ESTIMATE CLOSED LOOP ERROR X FOR VARIABLE SPEED : MATLAB Function  TreatAsAtomicUnit=on
  ESTIMATE CLOSED LOOP ERROR Y FOR VARIABLE SPEED : MATLAB Function  TreatAsAtomicUnit=on
  How much dx depends on x0 : Constant  Value=B_dx_versus_x0
  RealVsFakeWeight : Constant  Value=2
  RealVsFakeWeight1 : Constant  Value=2
  Sum : Sum  Inputs=|+-
  Sum1 : Sum  Inputs=|+-
  Terminator{2..7} (6 alike) : Terminator
  XY Foot Correction : Scope  NumInputPorts=2
      settings: YMin=-0~-0.1  YMax=0.04~0.125  SaveName=ScopeData39  SampleInput=on
  c_x_no_bias : Gain
  c_y_no_bias : Gain
  epsilon_x_no_bias : Gain
  epsilon_y_no_bias : Gain
  X Foot Correction [m] : Outport
  Y Foot Correction [m] : Outport  Port=2
  wires:
  RealVsFakeWeight1/1 -> ESTIMATE CLOSED LOOP ERROR Y FOR VARIABLE SPEED/5(W_real)
  Constant4/1 -> CLOSED LOOP COMPENSATION Y FOR VAIRABLE SPEED/6(B_cl)
  "target dY [m/s] "/1 -> Sum1/2, CLOSED LOOP COMPENSATION Y FOR VAIRABLE SPEED/5(dx_star)
  target dY History/1 -> ESTIMATE CLOSED LOOP ERROR Y FOR VARIABLE SPEED/4(dx_star_hist)
  Y Foot Correction History/1 -> ESTIMATE CLOSED LOOP ERROR Y FOR VARIABLE SPEED/2(delta_ux_hist)
  dY Takeoff History/1 -> ESTIMATE CLOSED LOOP ERROR Y FOR VARIABLE SPEED/3(dx_lift_hist)
  dY [m/s]/1 -> Sum1/1
  RealVsFakeWeight/1 -> ESTIMATE CLOSED LOOP ERROR X FOR VARIABLE SPEED/5(W_real)
  How much dx depends on x0/1 -> CLOSED LOOP COMPENSATION X FOR VAIRABLE SPEED/6(B_cl)
  Sum/1 -> CLOSED LOOP COMPENSATION X FOR VAIRABLE SPEED/4(delta_s_i)
  target dX [m/s]/1 -> Sum/2, CLOSED LOOP COMPENSATION X FOR VAIRABLE SPEED/5(dx_star)
  target dX History/1 -> ESTIMATE CLOSED LOOP ERROR X FOR VARIABLE SPEED/4(dx_star_hist)
  X Foot Correction History/1 -> ESTIMATE CLOSED LOOP ERROR X FOR VARIABLE SPEED/2(delta_ux_hist)
  dX Takeoff History/1 -> ESTIMATE CLOSED LOOP ERROR X FOR VARIABLE SPEED/3(dx_lift_hist)
  dX Touchdown History/1 -> ESTIMATE CLOSED LOOP ERROR X FOR VARIABLE SPEED/1(dx_land_hist)
  dX [m/s]/1 -> Sum/1
  dY Touchdown History/1 -> ESTIMATE CLOSED LOOP ERROR Y FOR VARIABLE SPEED/1(dx_land_hist)
  Sum1/1 -> CLOSED LOOP COMPENSATION Y FOR VAIRABLE SPEED/4(delta_s_i)
  CLOSED LOOP COMPENSATION X FOR VAIRABLE SPEED/1(delta_ux) -> XY Foot Correction/1, X Foot Correction [m]/1
  CLOSED LOOP COMPENSATION Y FOR VAIRABLE SPEED/1(delta_ux) -> XY Foot Correction/2, Y Foot Correction [m]/1
  ESTIMATE CLOSED LOOP ERROR X FOR VARIABLE SPEED/6(c_nb) -> c_x_no_bias/1
  ESTIMATE CLOSED LOOP ERROR X FOR VARIABLE SPEED/5(epsilon_0_nb) -> epsilon_x_no_bias/1
  ESTIMATE CLOSED LOOP ERROR X FOR VARIABLE SPEED/4(A_cl_nb) -> A_x_no_bias/1
  A_x_no_bias/1 -> Terminator5/1
  epsilon_x_no_bias/1 -> Terminator6/1
  c_x_no_bias/1 -> Terminator7/1
  A_y_no_bias/1 -> Terminator2/1
  epsilon_y_no_bias/1 -> Terminator3/1
  c_y_no_bias/1 -> Terminator4/1
  ESTIMATE CLOSED LOOP ERROR Y FOR VARIABLE SPEED/4(A_cl_nb) -> A_y_no_bias/1
  ESTIMATE CLOSED LOOP ERROR Y FOR VARIABLE SPEED/5(epsilon_0_nb) -> epsilon_y_no_bias/1
  ESTIMATE CLOSED LOOP ERROR Y FOR VARIABLE SPEED/6(c_nb) -> c_y_no_bias/1
  ESTIMATE CLOSED LOOP ERROR X FOR VARIABLE SPEED/3(c) -> "A, eps, c"/3, CLOSED LOOP COMPENSATION X FOR VAIRABLE SPEED/3(c)
  ESTIMATE CLOSED LOOP ERROR X FOR VARIABLE SPEED/2(epsilon_0) -> "A, eps, c"/2, CLOSED LOOP COMPENSATION X FOR VAIRABLE SPEED/2(epsilon)
  ESTIMATE CLOSED LOOP ERROR X FOR VARIABLE SPEED/1(A_cl) -> CLOSED LOOP COMPENSATION X FOR VAIRABLE SPEED/1(A_cl), "A, eps, c"/1
  ESTIMATE CLOSED LOOP ERROR Y FOR VARIABLE SPEED/3(c) -> CLOSED LOOP COMPENSATION Y FOR VAIRABLE SPEED/3(c)
  ESTIMATE CLOSED LOOP ERROR Y FOR VARIABLE SPEED/2(epsilon_0) -> CLOSED LOOP COMPENSATION Y FOR VAIRABLE SPEED/2(epsilon)
  ESTIMATE CLOSED LOOP ERROR Y FOR VARIABLE SPEED/1(A_cl) -> CLOSED LOOP COMPENSATION Y FOR VAIRABLE SPEED/1(A_cl)

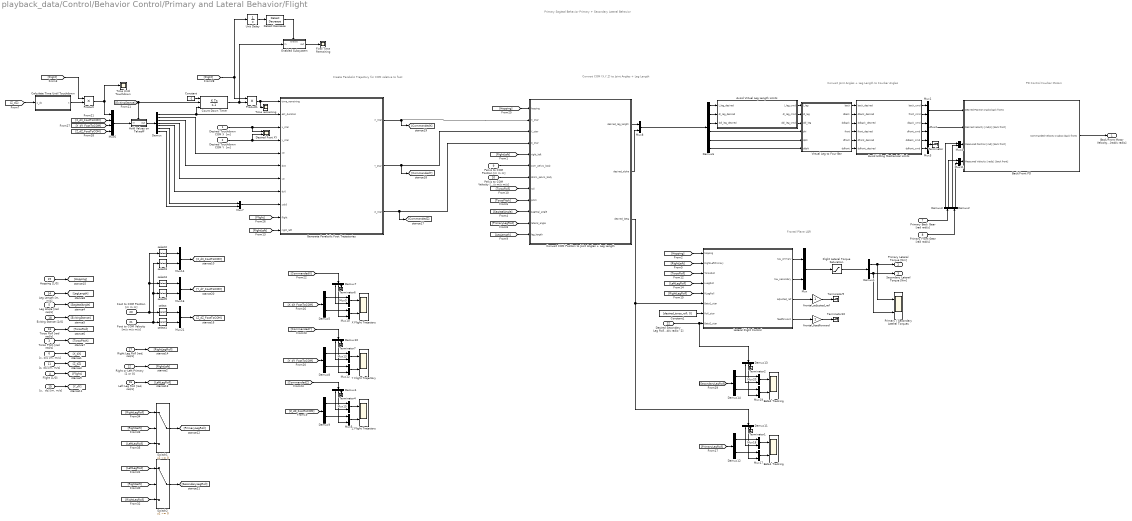
== system playback_data/Control/Behavior Control/Primary and Lateral Behavior/Flight ==
  note: Primary Sagittal Behavior
      | Primary + Secondary Lateral Behavior
  note: Create Parabolic
      | Trajectory for COM relative to foot
  note: Convert COM (X,Y,Z) to
      | Joint Angles + Leg Length
  note: Convert Joint Angles + Leg Length
      | to Fourbar Angles
  note: PD Control Fourbar Motors
  note: Frontal Plane LQR
  Desired Touchdown COM X  [m] : Inport
  Desired Touchdown COM Y  [m] : Inport  Port=2
  Torso Pitch [rad rad/s] : Inport  Port=3
  Flight [1/0] : Inport  Port=4
  Leg Angle [rad rad/s] : Inport  Port=5
  "[x, dx] [m, m/s]" : Inport  Port=6
  Primary Back Gear [rad rad/s] : Inport  Port=7
  Primary Front Gear [rad rad/s] : Inport  Port=8
  Pelvis to COM Position [m m m] : Inport  Port=9
  Pelvis to COM Velocity [m/s m/s m/s] : Inport  Port=10
  "[z, dz] [m, m/s]" : Inport  Port=11
  Right or Left Primary [1 or 0] : Inport  Port=12
  Torso Roll [rad rad/s] : Inport  Port=13
  "Leg Length [m, m/s]" : Inport  Port=14
  "[y,  dy] [m, m/s]" : Inport  Port=15
  "Left Leg Roll [rad, rad/s]" : Inport  Port=16
  "Right Leg Roll [rad, rad/s]" : Inport  Port=17
  Exiting Stance [1/0] : Inport  Port=18
  Hopping [1/0] : Inport  Port=19
  Foot to COM Position [m m m] : Inport  Port=20
  Foot to COM Velocity [m/s m/s m/s] : Inport  Port=21
  Desired Secondary Leg Roll [rad rad/s rad/s^2] : Inport  Port=22
  Avoid Hitting Mechanical Limits : MATLAB Function  TreatAsAtomicUnit=on
  Avoid Virtual Leg Length Limits : MATLAB Function  TreatAsAtomicUnit=on
  Back/Front PD : Subsystem
  Beta1 Tracking : Scope  NumInputPorts=2
      settings: YMin=1.3~-2  YMax=1.75~2.25  SaveName=ScopeData61  SampleInput=on
  Beta2 Tracking : Scope  NumInputPorts=2
      settings: YMin=1.3~-2  YMax=1.75~2.25  SaveName=ScopeData46  SampleInput=on
  Calculate Time Until Touchdown : MATLAB Function  TreatAsAtomicUnit=on
  Constant : Constant  Value=-1
  Constant1 : Constant  Value=[desired_torso_roll; 0]
  "Convert COM Position to Joint Angles + Leg Length " : MATLAB Function  TreatAsAtomicUnit=on
  Count Down Timer : DiscreteIntegrator  ExternalReset=rising  InitialConditionSource=external  InitialConditionSetting=State (most efficient)  SampleTime=sample_time  LimitOutput=on  LowerSaturationLimit=0
  Demux : Demux  Outputs=7
  Demux{1..3,5,8..9,12,14} (8 alike) : Demux  Outputs=2
  Demux{4,7,10..11,13} (5 alike) : Demux  Outputs=3
  Demux6 : Demux  Outputs=6
  Desired Foot XY : Scope  NumInputPorts=2
      settings: YMin=-1~-0.8  YMax=1~1.4  SaveName=ScopeData38  SampleInput=on
  Detect Decrease : simulink/Logic and Bit Operations/Detect Decrease  vinit=0.0  InputProcessing=Inherited  OutDataTypeStr=boolean
  Enabled Subsystem : Subsystem  TreatAsAtomicUnit=on
  Final Time Remaining : Scope
      settings: YMin=0  YMax=0.0275  SaveName=ScopeData51
  Flight Lateral Torque Saturation : Saturate  UpperLimit=HIP_MTR_MAX_CONT_TORQUE  LowerLimit=-HIP_MTR_MAX_CONT_TORQUE
      settings: AttributesFormatString=Top: %<UpperLimit>\nBottom: %<LowerLimit>
  Generate Parabolic Foot Trajectories : MATLAB Function  TreatAsAtomicUnit=on
  Hold Values on Takeoff : Subsystem
  Lateral Flight Control : MATLAB Function  TreatAsAtomicUnit=on
  Mux{,1..5,7..21} (21 alike) : Mux  Inputs=2
  Mux6 : Mux
  Primary / Secondary Lateral Torques : Scope  NumInputPorts=2
      settings: YMin=-1~-0.8  YMax=1~1.4  SaveName=ScopeData32  SampleInput=on
  Product : Product
  Product1 : Product
  Switch1 : Switch  Criteria=u2 ~= 0
  Switch2 : Switch  Criteria=u2 ~= 0
  Terminator{,1..2,4,6..7,9..10} (8 alike) : Terminator
  Time Until Touchdown : Scope
      settings: YMin=-0.125  YMax=0.175  SaveName=ScopeData37  SampleInput=on
  Time remaining : Scope
      settings: YMin=0  YMax=0.07  SaveName=ScopeData52
  Unit Delay : UnitDelay  SampleTime=-1
  Virtual Leg to Four Bar : MATLAB Function  TreatAsAtomicUnit=on
  X Flight Trajectory : Scope  NumInputPorts=2
      settings: YMin=-0.325~-3.25  YMax=0.225~2.25  SaveName=ScopeData3  SampleInput=on
  Y Flight Trajectory : Scope  NumInputPorts=2
      settings: YMin=-0.225~-2.25  YMax=0.2~1.25  SaveName=ScopeData4  SampleInput=on
  Z Flight Trajectory : Scope  NumInputPorts=2
      settings: YMin=0~-0.2  YMax=1.05~0.5  SaveName=ScopeData7  SampleInput=on
  frontal_adjusted_ref : Gain
  frontal_feedforward : Gain
  select : Selector  InputPortWidth=3  Indices=[3]
  select1 : Selector  InputPortWidth=3  Indices=[3]
  select2 : Selector  InputPortWidth=3  Indices=[1]
  select3 : Selector  InputPortWidth=3  Indices=[1]
  select4 : Selector  InputPortWidth=3  Indices=[2]
  select5 : Selector  InputPortWidth=3  Indices=[2]
  Back/Front Motor Velocity [rad/s rad/s] : Outport
  Primary Lateral Torque [Nm] : Outport  Port=2
  Secondary Lateral Torque [Nm] : Outport  Port=3
  wires:
  [RightLegRoll] -> Switch1/1
  [RightLeft] -> Switch1/2
  [LeftLegRoll] -> Switch1/3
  [RightLegRoll] -> Switch2/3
  [LeftLegRoll] -> Switch2/1
  [RightLeft] -> Switch2/2
  Switch2/1 -> [SecondaryLegRoll]
  Mux20/1 -> Beta2 Tracking/1
  Mux19/1 -> Beta2 Tracking/2
  Demux14/1 -> Mux20/1
  Demux14/2 -> Mux19/1
  Demux13/1 -> Mux20/2
  Demux13/2 -> Mux19/2
  [SecondaryLegRoll] -> Demux14/1
  Demux13/3 -> Terminator2/1
  [RightLeft] -> Generate Parabolic Foot Trajectories/11(right_left)
  Virtual Leg to Four Bar/1(back) -> Avoid Hitting Mechanical Limits/1(back_desired)
  Virtual Leg to Four Bar/2(dback) -> Avoid Hitting Mechanical Limits/2(dback_desired)
  Virtual Leg to Four Bar/3(ddback) -> Avoid Hitting Mechanical Limits/3(ddback_desired)
  Virtual Leg to Four Bar/4(front) -> Avoid Hitting Mechanical Limits/4(front_desired)
  Virtual Leg to Four Bar/5(dfront) -> Avoid Hitting Mechanical Limits/5(dfront_desired)
  Virtual Leg to Four Bar/6(ddfront) -> Avoid Hitting Mechanical Limits/6(ddfront_desired)
  Mux11/1 -> Back/Front PD/4(Measured Velocity [rad/s] [back front])
  Demux2/2 -> Mux11/2
  Mux4/1 -> Back/Front PD/3(Measured Position [rad] [back front])
  Mux1/1 -> Back/Front PD/1(Desired Position [rad] [back front])
  Demux3/2 -> Mux11/1
  Demux3/1 -> Mux4/1
  Avoid Hitting Mechanical Limits/2(front_cmd) -> Mux1/2
  Avoid Hitting Mechanical Limits/1(back_cmd) -> Mux1/1
  Demux2/1 -> Mux4/2
  Avoid Hitting Mechanical Limits/3(dback_cmd) -> Mux2/1
  Avoid Hitting Mechanical Limits/4(dfront_cmd) -> Mux2/2
  Avoid Hitting Mechanical Limits/5(ddback_cmd) -> Mux3/1
  Avoid Hitting Mechanical Limits/6(ddfront_cmd) -> Mux3/2
  Mux2/1 -> Back/Front PD/2(Desired Velocity [rad/s] [back front])
  Back/Front PD/1(Commanded Velocity [rad/s] [back front]) -> Back/Front Motor Velocity [rad/s rad/s]/1
  Primary Back Gear [rad rad/s]/1 -> Demux3/1
  Primary Front Gear [rad rad/s]/1 -> Demux2/1
  Demux/1 -> Count Down Timer/3, Generate Parabolic Foot Trajectories/2(est_duration)
  Mux7/1 -> Generate Parabolic Foot Trajectories/9(zdz0)
  Mux6/1 -> Hold Values on Takeoff/1(in)
  Hold Values on Takeoff/1(out) -> Demux/1
  [X_dX_FootToCOM] -> Mux6/2
  Generate Parabolic Foot Trajectories/1(X_star) -> [CommandedX], "Convert COM Position to Joint Angles + Leg Length "/2(X_star)
  Generate Parabolic Foot Trajectories/2(Y_star) -> "Convert COM Position to Joint Angles + Leg Length "/3(Y_star), [CommandedY]
  [RightLeft] -> "Convert COM Position to Joint Angles + Leg Length "/5(right_left)
  "Convert COM Position to Joint Angles + Leg Length "/2(desired_alpha) -> Mux8/2
  "Convert COM Position to Joint Angles + Leg Length "/1(desired_leg_length) -> Mux8/1
  Demux6/6 -> Virtual Leg to Four Bar/6(ddphi)
  Demux6/5 -> Virtual Leg to Four Bar/5(dphi)
  Demux6/4 -> Virtual Leg to Four Bar/4(phi)
  Mux8/1 -> Demux6/1
  Leg Angle [rad rad/s]/1 -> [SagittalAngle]
  [SagittalAngle] -> "Convert COM Position to Joint Angles + Leg Length "/10(sagittal_angle)
  Torso Pitch [rad rad/s]/1 -> [TorsoPitch]
  [TorsoPitch] -> "Convert COM Position to Joint Angles + Leg Length "/9(pitch)
  [PrimaryLegRoll] -> "Convert COM Position to Joint Angles + Leg Length "/11(lateral_angle)
  [LegLength] -> "Convert COM Position to Joint Angles + Leg Length "/12(leg_length)
  [TorsoRoll] -> "Convert COM Position to Joint Angles + Leg Length "/8(roll)
  Pelvis to COM Position [m m m]/1 -> "Convert COM Position to Joint Angles + Leg Length "/6(com_pelvis_body)
  Pelvis to COM Velocity [m/s m/s m/s]/1 -> "Convert COM Position to Joint Angles + Leg Length "/7(dcom_pelvis_body)
  Flight [1/0]/1 -> [Flight]
  [ExitingStance] -> Hold Values on Takeoff/Trigger, Count Down Timer/2
  "[x, dx] [m, m/s]"/1 -> [X_dX]
  Torso Roll [rad rad/s]/1 -> [TorsoRoll]
  "Leg Length [m, m/s]"/1 -> [LegLength]
  "[z, dz] [m, m/s]"/1 -> [Z_dZ]
  Desired Touchdown COM X  [m]/1 -> Desired Foot XY/1, Generate Parabolic Foot Trajectories/3(x_star)
  "[y,  dy] [m, m/s]"/1 -> [Y_dY]
  [Y_dY_FootToCOM] -> Mux6/3
  [Z_dZ] -> Calculate Time Until Touchdown/1(z_dz)
  Product/1 -> Time Until Touchdown/1, Mux6/1
  Avoid Virtual Leg Length Limits/1(l_leg_cmd) -> Virtual Leg to Four Bar/1(l_leg)
  Avoid Virtual Leg Length Limits/2(dl_leg_cmd) -> Virtual Leg to Four Bar/2(dl_leg)
  Avoid Virtual Leg Length Limits/3(ddl_leg_cmd) -> Virtual Leg to Four Bar/3(ddl_leg)
  Demux6/1 -> Avoid Virtual Leg Length Limits/1(l_leg_desired)
  Demux6/2 -> Avoid Virtual Leg Length Limits/2(dl_leg_desired)
  Demux6/3 -> Avoid Virtual Leg Length Limits/3(ddl_leg_desired)
  Desired Touchdown COM Y  [m]/1 -> Desired Foot XY/2, Generate Parabolic Foot Trajectories/4(y_star)
  [RightLeft] -> Lateral Flight Control/2(RightLeftPrimary)
  [TorsoRoll] -> Lateral Flight Control/3(TorsoRoll)
  Constant1/1 -> Lateral Flight Control/7(Roll_star)
  Lateral Flight Control/3(adjusted_ref) -> frontal_adjusted_ref/1
  Lateral Flight Control/4(feedforward) -> frontal_feedforward/1
  Lateral Flight Control/2(tau_secondary) -> Mux/2
  Lateral Flight Control/1(tau_primary) -> Mux/1
  "Left Leg Roll [rad, rad/s]"/1 -> [LeftLegRoll]
  [LeftLegRoll] -> Lateral Flight Control/4(LLegRoll)
  [RightLegRoll] -> Lateral Flight Control/5(RLegRoll)
  "Right Leg Roll [rad, rad/s]"/1 -> [RightLegRoll]
  Right or Left Primary [1 or 0]/1 -> [RightLeft]
  Switch1/1 -> [PrimaryLegRoll]
  Exiting Stance [1/0]/1 -> [ExitingStance]
  Demux1/1 -> Primary / Secondary Lateral Torques/1, Primary Lateral Torque [Nm]/1
  Demux1/2 -> Primary / Secondary Lateral Torques/2, Secondary Lateral Torque [Nm]/1
  Flight Lateral Torque Saturation/1 -> Demux1/1
  frontal_feedforward/1 -> Terminator10/1
  frontal_adjusted_ref/1 -> Terminator9/1
  [Hopping] -> "Convert COM Position to Joint Angles + Leg Length "/1(hopping)
  Mux/1 -> Flight Lateral Torque Saturation/1
  [Hopping] -> Lateral Flight Control/1(hopping)
  Hopping [1/0]/1 -> [Hopping]
  [Flight] -> Generate Parabolic Foot Trajectories/10(flight)
  Demux/2 -> Generate Parabolic Foot Trajectories/5(x0)
  Demux/3 -> Generate Parabolic Foot Trajectories/6(dx0)
  Demux/4 -> Generate Parabolic Foot Trajectories/7(y0)
  Demux/5 -> Generate Parabolic Foot Trajectories/8(dy0)
  Demux/6 -> Mux7/1
  Demux/7 -> Mux7/2
  select/1 -> Mux21/1
  select1/1 -> Mux21/2
  Mux21/1 -> [Z_dZ_FootToCOM]
  Mux15/1 -> Z Flight Trajectory/1
  Mux5/1 -> Z Flight Trajectory/2
  [Z_dZ_FootToCOM] -> Mux6/4
  [Z_dZ_FootToCOM] -> Demux9/1
  Demux9/1 -> Mux15/1
  Demux9/2 -> Mux5/1
  Demux4/1 -> Mux15/2
  Demux4/2 -> Mux5/2
  Demux4/3 -> Terminator4/1
  Mux9/1 -> X Flight Trajectory/1
  Mux10/1 -> X Flight Trajectory/2
  Demux5/1 -> Mux9/1
  Demux5/2 -> Mux10/1
  Demux7/1 -> Mux9/2
  Demux7/2 -> Mux10/2
  [X_dX_FootToCOM] -> Demux5/1
  Demux7/3 -> Terminator6/1
  Mux13/1 -> Y Flight Trajectory/1
  Mux12/1 -> Y Flight Trajectory/2
  Demux8/1 -> Mux13/1
  Demux8/2 -> Mux12/1
  Demux10/1 -> Mux13/2
  Demux10/2 -> Mux12/2
  [Y_dY_FootToCOM] -> Demux8/1
  Demux10/3 -> Terminator7/1
  [CommandedX] -> Demux7/1
  [CommandedY] -> Demux10/1
  [CommandedZ] -> Demux4/1
  Generate Parabolic Foot Trajectories/3(Z_star) -> "Convert COM Position to Joint Angles + Leg Length "/4(Z_star), [CommandedZ]
  Mux3/1 -> Terminator/1
  select2/1 -> Mux14/1
  select3/1 -> Mux14/2
  Mux14/1 -> [X_dX_FootToCOM]
  Foot to COM Position [m m m]/1 -> select4/1, select2/1, select/1
  Foot to COM Velocity [m/s m/s m/s]/1 -> select5/1, select3/1, select1/1
  select4/1 -> Mux16/1
  select5/1 -> Mux16/2
  Mux16/1 -> [Y_dY_FootToCOM]
  Calculate Time Until Touchdown/1(t) -> Product/2
  [Flight] -> Product/1
  Constant/1 -> Count Down Timer/1
  Count Down Timer/1 -> Enabled Subsystem/1(in), Product1/2
  Product1/1 -> Time remaining/1, Generate Parabolic Foot Trajectories/1(time_remaining)
  [Flight] -> Unit Delay/1, Product1/1
  Enabled Subsystem/1(out) -> Final Time Remaining/1
  Detect Decrease/1 -> Enabled Subsystem/Enable
  Unit Delay/1 -> Detect Decrease/1
  Mux18/1 -> Beta1 Tracking/1
  Mux17/1 -> Beta1 Tracking/2
  Demux12/1 -> Mux18/1
  Demux12/2 -> Mux17/1
  Demux11/1 -> Mux18/2
  Demux11/2 -> Mux17/2
  [PrimaryLegRoll] -> Demux12/1
  Demux11/3 -> Terminator1/1
  "Convert COM Position to Joint Angles + Leg Length "/3(desired_beta) -> Demux11/1, Lateral Flight Control/6(Beta1_star)
  Desired Secondary Leg Roll [rad rad/s rad/s^2]/1 -> Lateral Flight Control/8(Beta2_star), Demux13/1
